simulink model "QPSK_HW_SW"  (R2017b)
settings: Solver=FixedStepDiscrete  StartTime=0.0  StopTime=inf  RelTol=1e-3
PreLoadFcn:
  | % Ensure SDR libraries are added to path
  | dev = sdrdev('PicoZed SDR');
  | dev.setupSession
  | clear dev; % clean up
  | 
  | sdrzQPSKTxFPGA_params = zynqRadioQPSKTxFPGAAD9361AD9364SL_init;
  | rcRolloff = 0.5;
  | sdrzQPSKrxFPGA = zynqRadioQPSKRxFPGAAD9361AD9364SL_init(rcRolloff);
  | % Need preamble & data from CST's QPSK Tx HDL example
  | qpsktxhdl=commqpsktxhdl_init();
  | 
  | % ARM Tx message
  | txtstr = '*Zynq HW/SW Codesign*';
InitFcn:
  | sdrzQPSKTxFPGA_params = zynqRadioQPSKTxFPGAAD9361AD9364SL_init;
  | rcRolloff = 0.5;
  | sdrzQPSKrxFPGA = zynqRadioQPSKRxFPGAAD9361AD9364SL_init(rcRolloff);
  | % Need preamble & data from CST's QPSK Tx HDL example
  | qpsktxhdl=commqpsktxhdl_init();
  | 
  | if (numel(txtstr) > 24)
  |   error('txtstr message must be less than 24 characters');
  | end;
undefined symbols (not defined in the file or in its folder): msglen
libraries: hdlsllib x15, dspsigops x6, commsequence2 x2, commdigbbndpm3 x2, dspmlti4 x2, commrandsrc3 x1, commutil2 x1, simulink x1, dspmathops x1
(part 2 of 2)

== system QPSK_HW_SW/HDL_QPSK/HDLRxIPCore/HDLRx/Timing Recovery/Loop Filter/Digital Filter ==
  In1 : Inport
  Add2 : Sum  OutDataTypeStr=fixdt(1,40,33)
  Unit Delay1 : UnitDelay  SampleTime=-1
  Out1 : Outport
  wires:
  In1/1 -> Add2/2
  Add2/1 -> Unit Delay1/1, Out1/1
  Unit Delay1/1 -> Add2/1

== system QPSK_HW_SW/HDL_QPSK/HDLTxIPCore/HDLTx/Data Generation & Packetization/Data Source/HDL Data Scrambler ==
  note: HDL optimized scrambler, implementing the scrambler
      | polynomial [1 1 1 0 1], with initial states [0 0 0 0]
  Data_In : Inport
  Enable : EnablePort
  BIT_XOR : Logic  Operator=XOR  IconShape=distinctive  AllPortsSameDT=off  OutDataTypeStr=boolean
  BIT_XOR1 : Logic  Operator=XOR  IconShape=distinctive  AllPortsSameDT=off  OutDataTypeStr=boolean
  BIT_XOR2 : Logic  Operator=XOR  IconShape=distinctive  AllPortsSameDT=off  OutDataTypeStr=boolean
  p{1..4} (4 alike) : Delay  DelayLength=1
  Scrambled_Out : Outport  InitialOutput=0
  wires:
  BIT_XOR2/1 -> p1/1, Scrambled_Out/1
  p4/1 -> BIT_XOR/2
  p1/1 -> p2/1, BIT_XOR1/1
  BIT_XOR/1 -> BIT_XOR1/2
  p3/1 -> p4/1
  p2/1 -> p3/1, BIT_XOR/1
  BIT_XOR1/1 -> BIT_XOR2/2
  Data_In/1 -> BIT_XOR2/1

== matlab function QPSK_HW_SW/Descramble and Print/BitsToDecimal1 ==
  data: u input
function BitsToASCII(u)
%#codegen
% Convert bits to ASCII message.
% Convert binary-valued column vector to 7-bit decimal values.
w = [64 32 16 8 4 2 1]; % binary digit weighting
Nbits = numel(u);
Ny = Nbits/7;
y = zeros(1,Ny);
for i = 0:Ny-1
    y(i+1) = w*u(7*i+(1:7));
end

% replace the non-printable characters with "^" char(94) 
% to indicate an error 
y(y > 126)= 94; 
y(y < 32) = 94;
% Display ASCII message to command window
fprintf('%s\n',char(y));

== matlab function QPSK_HW_SW/HDL_QPSK/HDLTxIPCore/HDLTx/Data Generation & Packetization/PacketizerFSM ==
  data: reset_preamble output; load_preamble output; load_data output
function [reset_preamble,load_preamble, load_data] = PacketizerFSM()
%#codegen

persistent packState;
persistent stateCounter;

sType = numerictype(0,1,0);
cType = numerictype(0,8,0);

if isempty(packState)
    packState = fi(0,'numerictype',sType);
    stateCounter  = fi(0,'numerictype',cType);
end

Pack_Preamble = fi(0,'numerictype',sType);
Append_Data   = fi(1,'numerictype',sType);

switch(packState)
    case Pack_Preamble %% Pack_Preamble
        load_preamble  = true;
        reset_preamble = false;
        load_data     = false;
        
        if stateCounter == 25; %% preamble loaded
            packState(:) = 1;      %% move to data packing
            stateCounter(:) = 0;   %% reset counter
        else
            packState(:) = 0;      %% remain in preamble packing
            stateCounter(:) = stateCounter +1; %% increment preamble count
        end
        
    case Append_Data %% Append_Data
        load_preamble  = false;
        reset_preamble = true;
        load_data     = true;
        
        if stateCounter == 173 %% data loaded
            packState(:) = 0;      %% move to preamble packing
            stateCounter(:) = 0;   %% reset counter
        else
            packState(:) = 1;      %% remain in data loading
            stateCounter(:) = stateCounter +1; %% increment data count
        end
        
    otherwise
        load_preamble  = false;
        reset_preamble = false;
        load_data     = false;
        stateCounter(:) = 0;
end

== matlab function QPSK_HW_SW/HDL_QPSK/HDLRxIPCore/HDLRx/Data Decoding/MATLAB Function3 ==
  data: dvalid output; Freeze_MF_Conj output; enable input; MF_Conj input
function [dvalid,Freeze_MF_Conj] = fcn(enable,MF_Conj)
%#codegen

persistent state;
persistent counter;
persistent MF_Out_Reg;

if isempty(state);
    state      = false;
    counter    = uint8(0);
    MF_Out_Reg = complex(fi(0,1,16,10),fi(0,1,16,10));
end

Freeze_MF_Conj = MF_Out_Reg;

if state==false
    dvalid=false;
else %state==true
    dvalid=true;
    counter = counter-1;         
end


% state transition
if state==false && enable==true
    state=true;
    counter=uint8(100);
    MF_Out_Reg=MF_Conj;
elseif state==true && counter==0
    if enable==true % packages come back-to-back
        state      = true;
        counter    = uint8(100);
        MF_Out_Reg = MF_Conj;
    else
        state = false;    
    end
end

== matlab function QPSK_HW_SW/Descramble and Print/DataFramer ==
  data: dataIn input; dataOut output
function dataOut = fcn(dataIn)
%#codegen


nData = 2*numel(dataIn);

b1 = real(dataIn);
b2 = imag(dataIn);

dataOut = logical(reshape([b1,b2]',nData,1));

== matlab function QPSK_HW_SW/HDL_QPSK/HDLRxIPCore/HDLRx/Timing Recovery/Interpolation Control ==
  data: Delta input; Underflow output; mu output
function [Underflow, mu] = Interpolation_ctrl(Delta)
% Implementation of modulo-1 counter for interpolation control listed in
% Figure 8.4.19 of "Digital Communications - A Discrete-Time Approach"
% by Michael Rice. See design details in Chapter 8.4.3 of the same book.
% 
% Input:
%   Delta - Loop filter output. If loop is in lock, delta would be small
% Output:
%   Underflow - Indicator of counter underflow. This is the strobe signal
%               for downstream processing
%   mu - Difference between actual sampling instant and the optimal instant,
%        between zero and one
%#codegen

% delay1 - Counter value delayed by 1 sample
% Regtemp - The estimated timing error normalized by half QPSK symbols

persistent delay1 Regtemp;  
if isempty(delay1)
    delay1  = fi(0,1,11,10);
    Regtemp = fi(0,1,11,10);
end

mask = fi(1-2^(-10),1,11,10);

counter = bitand(mask,delay1)-Delta-fi(0.5,1,11,10); % decrementing counter
% if delay1 is a nonnegative number, 
% then mod(delay1,1) equals the fractional part of delay1

if counter < 0
    Underflow = true;
    Regtemp = bitshift(bitand(mask,delay1),1);     
else
    Underflow = false;
end

mu = Regtemp;

% Update delay buffer
%delay1 = counter;
if counter<0
    delay1 = fi(counter+1,1,11,10); %make sure delay1 is nonnegative
else
    delay1 = fi(counter,1,11,10);
end

== matlab function QPSK_HW_SW/HDL_QPSK/HDLRxIPCore/HDLRx/Timing Recovery/Timing Error Detector ==
  data: In input; strobe input; e output
function e = TED(In, strobe)
% Zero-Crossing Timing Error Detector. See "Zero-Crossing Timing Error
% Detector" section in Chapter 8.4.1 of "Digital Communications - A
% Discrete-Time Approach" by Michael Rice. For bit stuffing/stripping
% details, see page 490-494 of the same book.
%
% Input: 
%   In - Input samples, interpolation result
%   strobe - Signal to enable timing error calculation
% Output:
%   e - Timing error
%#codegen

persistent delay1_R delay1_I delay2_R delay2_I delayStrobe; 
% Input delayed by one and 2 samples, and
% Enable signal delayed by one sample
if isempty(delay1_R)    
    delay1_R=fi(0,1,16,10);
    delay1_I=fi(0,1,16,10);
    delay2_R=fi(0,1,16,10);
    delay2_I=fi(0,1,16,10);    
    delayStrobe = false;
end

In_Real = real(In);
In_Imag = imag(In);

if strobe==true && delayStrobe~=strobe
    if ( bitget(delay2_R,16)==bitget(In_Real,16) )         
        OP1=fi(0,1,16,10);
    elseif bitget(delay2_R,16)==true         
        OP1=fi(-1*bitshift(delay1_R,1),1,16,10);
    else        
        OP1=fi(bitshift(delay1_R,1),1,16,10);
    end
    
    if ( bitget(delay2_I,16)==bitget(In_Imag,16) )        
        OP2=fi(0,1,16,10);
    elseif bitget(delay2_I,16)==true        
        OP2=fi(-1*bitshift(delay1_I,1),1,16,10);
    else        
        OP2=fi(bitshift(delay1_I,1),1,16,10);
    end
else
    OP1=fi(0,1,16,10);
    OP2=fi(0,1,16,10);
end

e = fi(OP1+OP2,1,16,10);


if delayStrobe~=strobe
    % Shift contents in delay register
    delay2_R = delay1_R;
    delay1_R = In_Real;
    delay2_I = delay1_I;
    delay1_I = In_Imag;
elseif strobe==true
    % Two consecutive high strobes
    delay2_R = fi(0,1,16,10); % Stuff missing sample
    delay1_R = In_Real; 
    delay2_I = fi(0,1,16,10); % Stuff missing sample
    delay1_I = In_Imag; 
end

% If both current and previous enable signals are 0, skip current sample
% and keep the delayed signals unchanged. (Bit stripping)
delayStrobe = strobe;

== matlab function QPSK_HW_SW/HDL_QPSK/HDLRxIPCore/HDLRx/Fine Frequency Compensation/MATLAB Function1 ==
  data: In input; e output
function e  = PED(In)
% Input:
%   In - Input samples, oversampled by two
% Output:
%   e - Phase error
% PED implements 
% e = sign(real(In)).*imag(In) - sign(imag(In)).*real(In);

%#codegen

OP2 = real(In);
OP1 = imag(In);

Real = OP2;
Imag = OP1;

if (bitget(Real,16)==true) % real component is negative
    OP1 = fi(-Imag,1,16,14);
end
if (bitget(Imag,16)==true) % imaginary component is negative
    OP2 = fi(-Real,1,16,14);
end

e= fi(OP1-OP2,1,16,14);

%e = sign(real(In)).*imag(In) - sign(imag(In)).*real(In);
